simulink model "glideslope_flare"  (R2020a)
settings: Solver=FixedStepAuto  StartTime=0.0  StopTime=100  FixedStep=0.001  RelTol=1e-3
values from neighbouring files (symbols this model uses):
  A = [-0.0291    2.1300  -32.1700   -2.8952    0.0001 ... (first row only)    [glideslope_flare_params.m]
  B = [ 0.0045    0.0015 ... (first row only)    [glideslope_flare_params.m]
  C = [1.0000         0         0         0         0 ... (first row only)    [glideslope_flare_params.m]
  D = zeros(5,2)    [glideslope_flare_params.m]
undefined symbols (not defined in the file or in its folder): alpha0, de0, dt0, h0, q0, theta0, V0
libraries: simulink x2
settings Model: Creator=Pjotr  LastModifiedBy=Pjotr

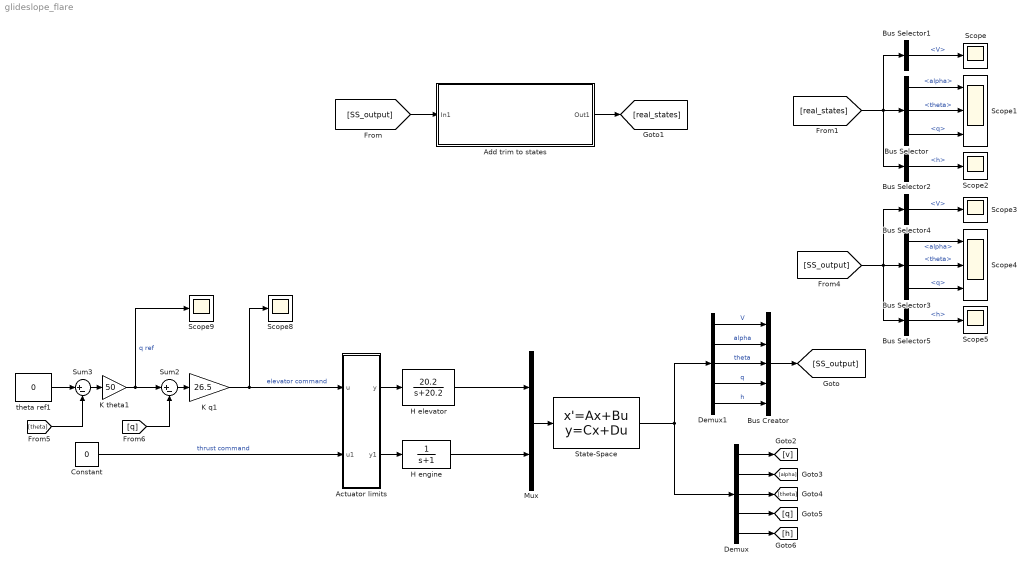
== system glideslope_flare ==
  Actuator limits : Subsystem
  Add trim to states : Subsystem
  Bus Creator : BusCreator  Inputs=5
  Bus Selector : BusSelector  OutputSignals=alpha,theta,q
  Bus Selector1 : BusSelector  OutputSignals=V
  Bus Selector2 : BusSelector  OutputSignals=h
  Bus Selector3 : BusSelector  OutputSignals=alpha,theta,q
  Bus Selector4 : BusSelector  OutputSignals=V
  Bus Selector5 : BusSelector  OutputSignals=h
  Constant : Constant  Value=0
  Demux : Demux  Outputs=5
  Demux1 : Demux  Outputs=5
  H elevator : TransferFcn  Numerator=20.2  Denominator=[1 20.2]
  H engine : TransferFcn  Denominator=[1 1]
  K q1 : Gain  Gain=26.5
  K theta1 : Gain  Gain=50
  Mux : Mux  Inputs=2
  Scope{,2..3,5,8..9} (6 alike) : Scope
  Scope1 : Scope  NumInputPorts=3
  Scope4 : Scope  NumInputPorts=3
  State-Space : StateSpace  A=A  B=B  C=C  D=D  InitialCondition=0
  Sum2 : Sum  Inputs=|+-
  Sum3 : Sum  Inputs=|+-
  theta ref1 : Constant  Value=0
  wires:
  [SS_output] -> Add trim to states/1(In1)
  Add trim to states/1(Out1) -> [real_states]
  [real_states] -> Bus Selector2/1, Bus Selector/1, Bus Selector1/1
  Bus Selector/1 -> Scope1/1  "<alpha>"
  Bus Selector/2 -> Scope1/2  "<theta>"
  Bus Selector/3 -> Scope1/3  "<q>"
  Bus Selector1/1 -> Scope/1  "<V>"
  Mux/1 -> State-Space/1
  Bus Selector2/1 -> Scope2/1  "<h>"
  State-Space/1 -> Demux1/1, Demux/1
  Actuator limits/1(y) -> H elevator/1
  H elevator/1 -> Mux/1
  H engine/1 -> Mux/2
  Actuator limits/2(y1) -> H engine/1
  Constant/1 -> Actuator limits/2(u1)  "thrust command"
  Demux/1 -> [v]
  Demux/2 -> [alpha]
  Demux/3 -> [theta]
  Demux/4 -> [q]
  Demux/5 -> [h]
  Bus Selector3/1 -> Scope4/1  "<alpha>"
  Bus Selector3/3 -> Scope4/3  "<q>"
  [SS_output] -> Bus Selector4/1, Bus Selector5/1, Bus Selector3/1
  Bus Selector4/1 -> Scope3/1  "<V>"
  Bus Selector5/1 -> Scope5/1  "<h>"
  Bus Selector3/2 -> Scope4/2  "<theta>"
  Demux1/1 -> Bus Creator/1  "V"
  Demux1/2 -> Bus Creator/2  "alpha"
  Demux1/3 -> Bus Creator/3  "theta"
  Demux1/5 -> Bus Creator/5  "h"
  Demux1/4 -> Bus Creator/4  "q"
  Bus Creator/1 -> [SS_output]
  K q1/1 -> Actuator limits/1(u), Scope8/1  "elevator command"
  Sum2/1 -> K q1/1
  [q] -> Sum2/2
  K theta1/1 -> Sum2/1, Scope9/1  "q ref"
  Sum3/1 -> K theta1/1
  theta ref1/1 -> Sum3/1
  [theta] -> Sum3/2

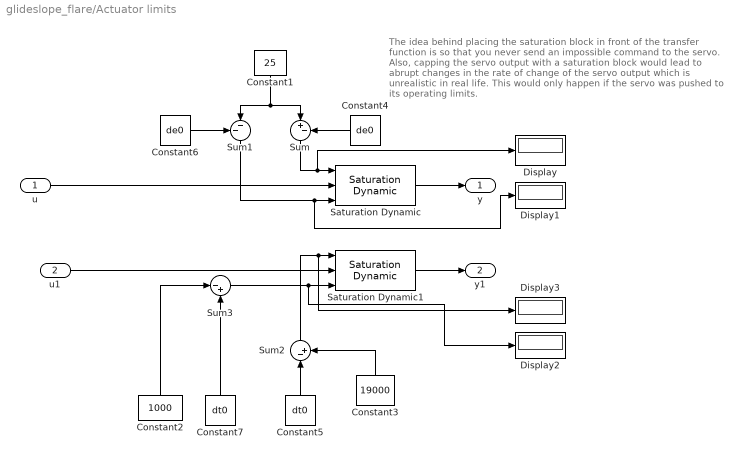
== system glideslope_flare/Actuator limits ==
  note: The idea behind placing the saturation block in front of
      | the transfer function is so that you never send an impossible
      | command to the servo. Also, capping the servo output with
      | a saturation block would lead to abrupt changes in the rate of change
      | of the servo output which is unrealistic in real life. This would only
      | happen if the servo was pushed to its operating limits.
  u : Inport
  u1 : Inport  Port=2
  Constant1 : Constant  Value=25
  Constant2 : Constant  Value=1000
  Constant3 : Constant  Value=19000
  Constant4 : Constant  Value=de0
  Constant5 : Constant  Value=dt0
  Constant6 : Constant  Value=de0
  Constant7 : Constant  Value=dt0
  Display{,1..3} (4 alike) : Display
  Saturation Dynamic : simulink/Discontinuities/Saturation Dynamic  OutMin=[]  OutMax=[]  OutDataTypeStr=Inherit: Same as second input  OutDataType=fixdt(1, 16)  OutScaling=2^-10  DoSatur=off
  Saturation Dynamic1 : simulink/Discontinuities/Saturation Dynamic  OutMin=[]  OutMax=[]  OutDataTypeStr=Inherit: Same as second input  OutDataType=fixdt(1, 16)  OutScaling=2^-10  DoSatur=off
  Sum : Sum  Inputs=|+-
  Sum1 : Sum  Inputs=--|
  Sum2 : Sum  Inputs=|-+
  Sum3 : Sum  Inputs=|-+
  y : Outport
  y1 : Outport  Port=2
  wires:
  Constant6/1 -> Sum1/1
  Constant5/1 -> Sum2/1
  Constant3/1 -> Sum2/2
  Constant1/1 -> Sum/1, Sum1/2
  Constant7/1 -> Sum3/2
  Sum3/1 -> Display2/1, Saturation Dynamic1/3
  Sum2/1 -> Display3/1, Saturation Dynamic1/1
  Saturation Dynamic/1 -> y/1
  Sum1/1 -> Display1/1, Saturation Dynamic/3
  Sum/1 -> Display/1, Saturation Dynamic/1
  Constant4/1 -> Sum/2
  Constant2/1 -> Sum3/1
  u1/1 -> Saturation Dynamic1/2
  u/1 -> Saturation Dynamic/2
  Saturation Dynamic1/1 -> y1/1

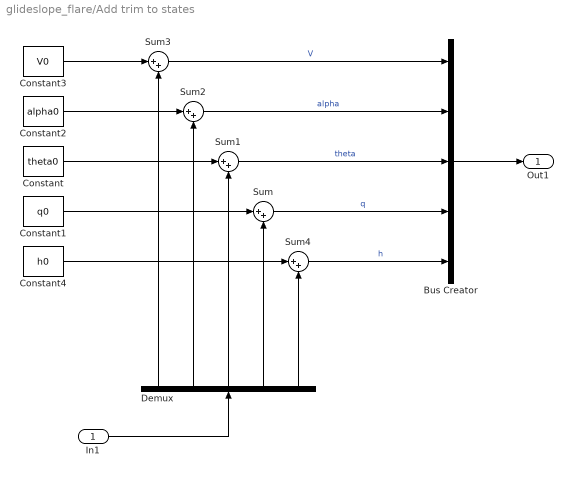
== system glideslope_flare/Add trim to states ==
  In1 : Inport
  Bus Creator : BusCreator  Inputs=5
  Constant : Constant  Value=theta0
  Constant1 : Constant  Value=q0
  Constant2 : Constant  Value=alpha0
  Constant3 : Constant  Value=V0
  Constant4 : Constant  Value=h0
  Demux : Demux  Outputs=5
  Sum{,1..4} (5 alike) : Sum  Inputs=|++
  Out1 : Outport
  wires:
  Sum/1 -> Bus Creator/4  "q"
  In1/1 -> Demux/1
  Constant3/1 -> Sum3/1
  Constant/1 -> Sum1/1
  Demux/3 -> Sum1/2
  Demux/2 -> Sum2/2
  Sum3/1 -> Bus Creator/1  "V"
  Constant1/1 -> Sum/1
  Sum1/1 -> Bus Creator/3  "theta"
  Constant2/1 -> Sum2/1
  Demux/4 -> Sum/2
  Demux/1 -> Sum3/2
  Sum2/1 -> Bus Creator/2  "alpha"
  Bus Creator/1 -> Out1/1
  Demux/5 -> Sum4/2
  Constant4/1 -> Sum4/1
  Sum4/1 -> Bus Creator/5  "h"
